simulink model "ativa_3W_R150"  (Simulink 10.1)
settings: Solver=ode23t  StartTime=0.0  StopTime=0.1  RelTol=1e-3  EnableMultiTasking=on
libraries: powerlib x8, powerlib_extras x2
settings Model: Creator=alunos  LastModifiedBy=victo
settings DataIOCC: LimitDataPoints=on  SignalLoggingSaveFormat=ModelDataLogs
settings OptimizationCC: ExpressionDepthLimit=2147483647
settings DebuggingCC: SolverPrmCheckMsg=warning  FcnCallInpInsideContextMsg=warning  StateNameClashWarn=warning

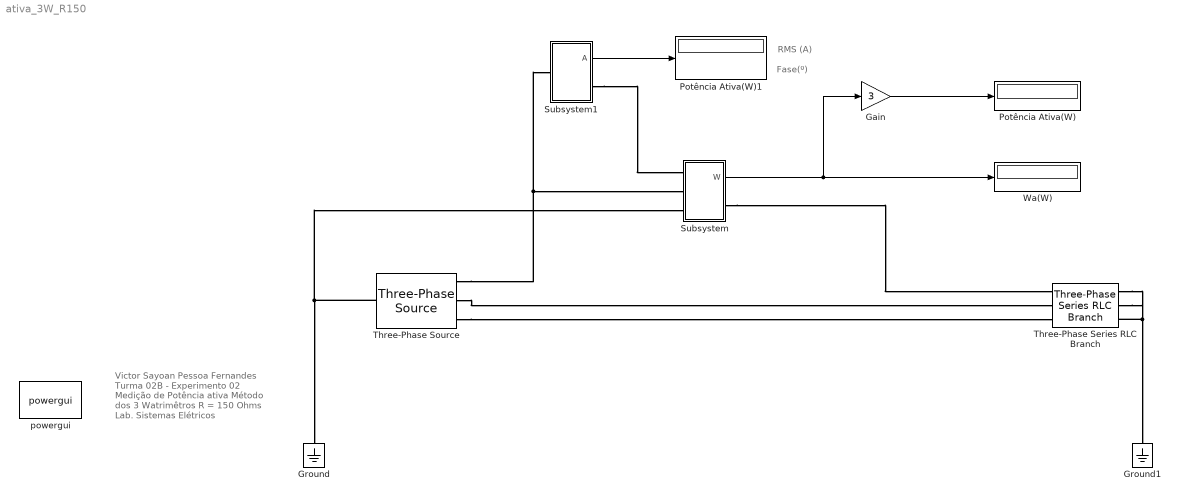
== system ativa_3W_R150 ==
  note: RMS (A)
  note: Fase(º)
  note: Victor Sayoan Pessoa Fernandes
      | Turma 02B - Experimento 02
      | Medição de Potência ativa
      | Método dos 3 Watrimêtros
      | R = 150 Ohms
      | Lab. Sistemas Elétricos
  Gain : Gain  Gain=3
  Ground : powerlib/Elements/Ground  LConnTagsString=a
  Ground1 : powerlib/Elements/Ground  LConnTagsString=a
  Potência Ativa(W) : Display
  Potência Ativa(W)1 : Display
  Subsystem : Subsystem
  Subsystem1 : Subsystem
  Three-Phase Series RLC Branch : powerlib/Elements/Three-Phase Series RLC Branch  LConnTagsString=A|B|C  RConnTagsString=A|B|C  BranchType=RL  Resistance=150  Inductance=300e-3  Capacitance=1e-6  Measurements=None
  Three-Phase Source : powerlib/Electrical Sources/Three-Phase Source  InternalConnection=Yn  VoltagePhases=off  Voltage=220  PhaseAngle=90  Voltage_phases=[25e3 25e3 25e3]/sqrt(3)  PhaseAngles_phases=[0 -120 +120]  Frequency=60  NonIdealSource=on  SpecifyImpedance=off  Resistance=0.001  Inductance=0  ShortCircuitLevel=100e6  BaseVoltage=25e3  XRratio=7  BusType=swing  Pref=0  Qref=0  Prefabc=[10e3, 10e3, 10e3]  Qrefabc=[0, 0, 0]  Qmin=-inf  Qmax=inf
  Wa(W) : Display
  powergui : powerlib/powergui  Priority=1  SimulationMode=Continuous  SampleTime=50e-6  frequency=60  Iterations=50  frequencyindice=60  Pbase=100e6  ErrMax=1e-4  UnitsV=kV  UnitsW=MW  buscounter=0  FunctionMessages=off  echomessages=off  EnableUseOfTLC=off  CurrentSourceSwitches=on  DisableSnubberDevices=off  DisableRonSwitches=off  DisableVfSwitches=off  DisplayEquations=off  AutomaticDiscreteSolvers=off  SolverType=Tustin/Backward Euler (TBE)  Interpol=off  ExternalGateDelay=off  methode=off  Ts=100  x0status=blocks  SPID=off  SwTol=0  HookPort=off  NonlinearTolerance=1e-4  nMaxIteration=100  ContinueOnMaxIteration=off  RestoreLinks=warning  ResistiveCurrentMeasurement=off  Frange=[0:2:500]  Ylog=off  Xlog=on  ShowGrid=off  save=off  variable=ZData  structure=0  ZoomFFT=off  StartTime=0.0  cycles=1  DisplayStyle=1  fundamental=60  FreqAxis=off  MaxFrequency=1000  frequencyindicesteady=1  RmsSteady=1  display=off
  wires:
  Subsystem/1(W) -> Wa(W)/1, Gain/1
  Gain/1 -> Potência Ativa(W)/1
  Subsystem1/1(A) -> Potência Ativa(W)1/1
  connections:
  Three-Phase Source/LConn1 -- Ground/LConn1 -- Subsystem/LConn3
  Three-Phase Series RLC Branch/RConn1 -- Three-Phase Series RLC Branch/RConn2 -- Three-Phase Series RLC Branch/RConn3 -- Ground1/LConn1
  Three-Phase Source/RConn2 -- Three-Phase Series RLC Branch/LConn2
  Three-Phase Source/RConn3 -- Three-Phase Series RLC Branch/LConn3
  Subsystem/RConn1 -- Three-Phase Series RLC Branch/LConn1
  Three-Phase Source/RConn1 -- Subsystem1/LConn1 -- Subsystem/LConn2
  Subsystem1/RConn1 -- Subsystem/LConn1

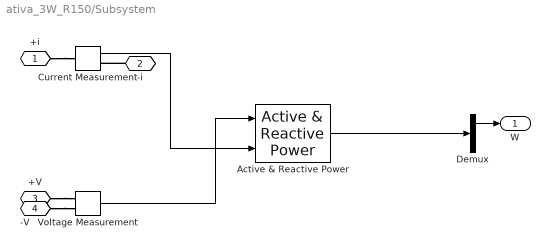
== system ativa_3W_R150/Subsystem ==
  Active & Reactive Power : powerlib_extras/Measurements/Active & Reactive Power  f1=60
      settings: SourceProductBaseCode=PS
  Current Measurement : powerlib/Measurements/Current Measurement  PhasorSimulation=off  OutputType=Complex  PSBequivalent=0
  Demux : Demux  Outputs=2
  Voltage Measurement : powerlib/Measurements/Voltage Measurement  PhasorSimulation=off  OutputType=Complex  PSBequivalent=0
  +i : PMIOPort  Side=Left
  -i : PMIOPort  Port=2  Side=Right
  +V : PMIOPort  Port=3  Side=Left
  -V : PMIOPort  Port=4  Side=Left
  W : Outport
  wires:
  Current Measurement/1 -> Active & Reactive Power/2
  Voltage Measurement/1 -> Active & Reactive Power/1
  Active & Reactive Power/1 -> Demux/1
  Demux/1 -> W/1
  connections:
  +i/RConn1 -- Current Measurement/LConn1
  -i/RConn1 -- Current Measurement/RConn1
  +V/RConn1 -- Voltage Measurement/LConn1
  -V/RConn1 -- Voltage Measurement/LConn2

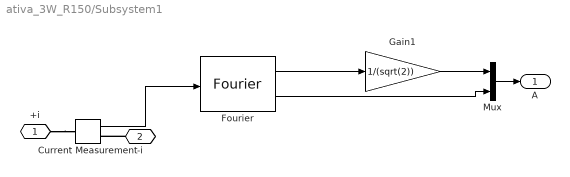
== system ativa_3W_R150/Subsystem1 ==
  Current Measurement : powerlib/Measurements/Current Measurement  PhasorSimulation=off  OutputType=Complex  PSBequivalent=0
  Fourier : powerlib_extras/Measurements/Fourier  f1=60  n=1
      settings: SourceProductBaseCode=PS
  Gain1 : Gain  Gain=1/(sqrt(2))
  Mux : Mux  Inputs=2
  +i : PMIOPort  Side=Left
  -i : PMIOPort  Port=2  Side=Right
  A : Outport
  wires:
  Current Measurement/1 -> Fourier/1
  Fourier/1 -> Gain1/1
  Gain1/1 -> Mux/1
  Fourier/2 -> Mux/2
  Mux/1 -> A/1
  connections:
  +i/RConn1 -- Current Measurement/LConn1
  -i/RConn1 -- Current Measurement/RConn1
